simulink model "progetto3Tenzo"  (Simulink 7.9)
settings: Solver=ode23s  StartTime=0.0  StopTime=100  RelTol=1e-3
values from neighbouring files (symbols this model uses):
  AMI = AK1    [AstaTenzo.m]    (also in BoundTenzo.m)
  AMin = [ ... (first row only)    [AstaTenzo.m]    (also in BoundTenzo.m; RiduzioneModello1_15.m)
  Aoss = AMin-V*ClocalMin    [AstaTenzo.m]    (also in BoundTenzo.m; RiduzioneModello1_15.m)
  BMI = BK1    [AstaTenzo.m]    (also in BoundTenzo.m)
  Bmod = [M BMin]    [AstaTenzo.m]    (also in BoundTenzo.m)
  Boss = [BMin-V*D V M-V*N]    [AstaTenzo.m]    (also in BoundTenzo.m; RiduzioneModello1_15.m = [BMin-V*D V])
  ClocalMin = [ ... (first row only)    [AstaTenzo.m]    (also in BoundTenzo.m; RiduzioneModello1_15.m)
  CMI = eye(q*mu)    [AstaTenzo.m]    (also in BoundTenzo.m)
  Coss = eye(n)    [AstaTenzo.m]    (also in BoundTenzo.m; RiduzioneModello1_15.m = eye(size(AMin)))
  DMI = zeros(q*mu,q)    [AstaTenzo.m]    (also in BoundTenzo.m)
  Dmod = [N D]    [AstaTenzo.m]    (also in BoundTenzo.m)
  Doss = zeros(size(Boss))    [AstaTenzo.m]    (also in BoundTenzo.m; RiduzioneModello1_15.m)
  F1 = F(:,size(AMin,1)+1:size(F,2))    [AstaTenzo.m]    (also in BoundTenzo.m)
  F2 = F(:,1:size(AMin,1))    [AstaTenzo.m]    (also in BoundTenzo.m)
  omega = 0.5    [AstaTenzo.m]    (also in BoundTenzo.m = logspace(-2,1,150); LTR_Tenzo.m = logspace(-2,3); Tenzo1_05.m = 4)
libraries: simulink x1
settings Model: Creator=danilo  LastModifiedBy=userk
settings DebuggingCC: FcnCallInpInsideContextMsg=Use local settings
settings GRTTargetCC: CombineOutputUpdateFcns=off  GRTInterface=on

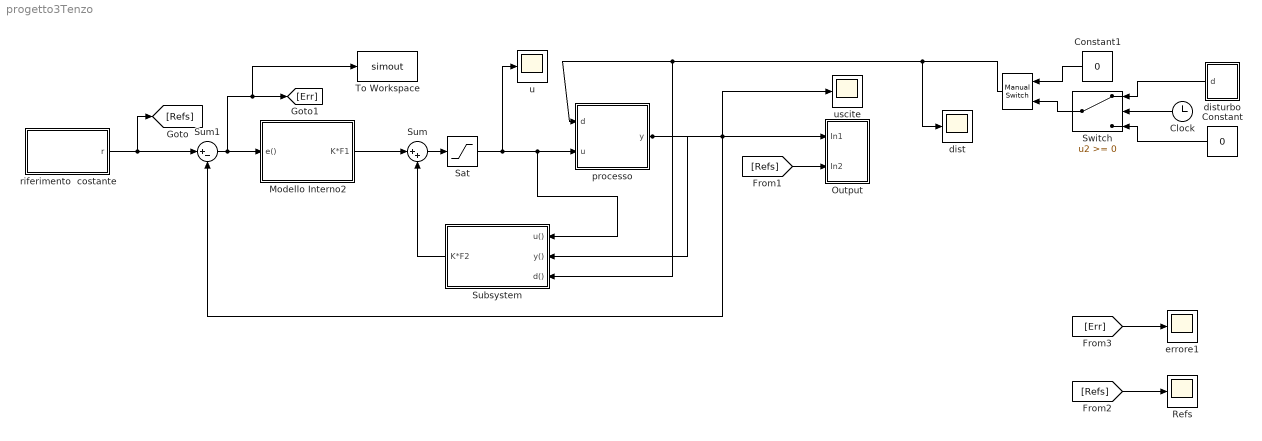
== system progetto3Tenzo ==
  " " : simulink/Signal Routing/Manual Switch  sw=0  action=0  varsize=off
  Clock : Clock
  Constant : Constant  Value=0
  Constant1 : Constant  Value=0
  Modello Interno2 : Subsystem
  Output : Subsystem
  Refs : Scope
  Sat : Saturate  UpperLimit=60  LowerLimit=-60
  Subsystem : Subsystem
  Sum : Sum  Inputs=|++
  Sum1 : Sum  Inputs=|+-
  Switch : Switch
  To Workspace : ToWorkspace  VariableName=simout  SampleTime=-1  SaveFormat=Structure
  dist : Scope
      settings: SaveName=ScopeData5
  disturbo : Subsystem
  errore1 : Scope
      settings: SaveName=ScopeData8
  processo : Subsystem
  riferimento  costante : Subsystem
  u : Scope
      settings: SaveName=ScopeData3
  uscite : Scope
      settings: SaveName=ScopeData2
  wires:
  riferimento  costante/1(r) -> Sum1/1, [Refs]
  processo/1(y) -> Sum1/2, Output/1(In1), uscite/1, Subsystem/2(y())
  Subsystem/1(K*F2) -> Sum/2
  Sum/1 -> Sat/1
  Sum1/1 -> To Workspace/1, [Err], Modello Interno2/1(e())
  [Refs] -> Output/2(In2)
  [Refs] -> Refs/1
  [Err] -> errore1/1
  Clock/1 -> Switch/2
  disturbo/1(d) -> Switch/1
  Constant/1 -> Switch/3
  Sat/1 -> processo/2(u), Subsystem/1(u()), u/1
  Switch/1 -> " "/2
  Constant1/1 -> " "/1
  " "/1 -> dist/1, processo/1(d), Subsystem/3(d())
  Modello Interno2/1(K*F1) -> Sum/1

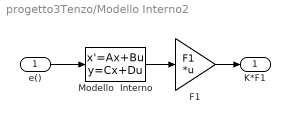
== system progetto3Tenzo/Modello Interno2 ==
  e() : Inport
  F1 : Gain  Gain=F1  Multiplication=Matrix(K*u) (u vector)
  Modello  Interno : StateSpace  A=AMI  B=BMI  C=CMI  D=DMI
  K*F1 : Outport
  wires:
  Modello  Interno/1 -> F1/1
  e()/1 -> Modello  Interno/1
  F1/1 -> K*F1/1

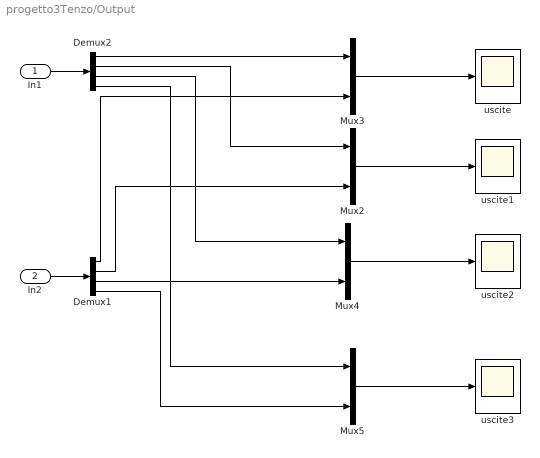
== system progetto3Tenzo/Output ==
  In1 : Inport
  In2 : Inport  Port=2
  Demux1 : Demux
  Demux2 : Demux
  Mux{2..5} (4 alike) : Mux  Inputs=2
  uscite{,1..3} (4 alike) : Scope
      uscite settings: TickLabels=on  YMin=-3.5  YMax=7
      uscite1 settings: TickLabels=on  TimeRange=30  YMin=0.75  YMax=4.25  SaveName=ScopeData4
      uscite2 settings: TickLabels=on  YMin=0.75  YMax=4.25  SaveName=ScopeData6
      uscite3 settings: TickLabels=on  YMin=0.75  YMax=4.25  SaveName=ScopeData7
  wires:
  Demux1/1 -> Mux3/2
  In2/1 -> Demux1/1
  In1/1 -> Demux2/1
  Mux3/1 -> uscite/1
  Demux2/1 -> Mux3/1
  Mux2/1 -> uscite1/1
  Demux2/2 -> Mux2/1
  Mux4/1 -> uscite2/1
  Demux2/3 -> Mux4/1
  Mux5/1 -> uscite3/1
  Demux2/4 -> Mux5/1
  Demux1/2 -> Mux2/2
  Demux1/3 -> Mux4/2
  Demux1/4 -> Mux5/2

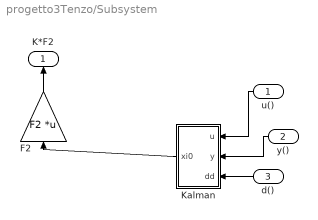
== system progetto3Tenzo/Subsystem ==
  u() : Inport
  y() : Inport  Port=2
  d() : Inport  Port=3
  F2 : Gain  Gain=F2  Multiplication=Matrix(K*u) (u vector)
  Kalman : Subsystem
  K*F2 : Outport
  wires:
  Kalman/1(xi0) -> F2/1
  u()/1 -> Kalman/1(u)
  y()/1 -> Kalman/2(y)
  d()/1 -> Kalman/3(dd)
  F2/1 -> K*F2/1

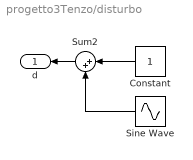
== system progetto3Tenzo/disturbo ==
  Constant : Constant
  Sine Wave : Sin  Amplitude=3  Frequency=omega  SampleTime=0
  Sum2 : Sum  Inputs=|++
  d : Outport
  wires:
  Sine Wave/1 -> Sum2/2
  Constant/1 -> Sum2/1
  Sum2/1 -> d/1

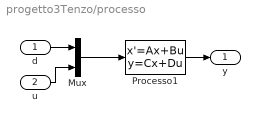
== system progetto3Tenzo/processo ==
  d : Inport
  u : Inport  Port=2
  Mux : Mux  Inputs=[1 4]
  Processo1 : StateSpace  A=AMin  B=Bmod  C=ClocalMin  D=Dmod
  y : Outport
  wires:
  Mux/1 -> Processo1/1
  d/1 -> Mux/1
  Processo1/1 -> y/1
  u/1 -> Mux/2

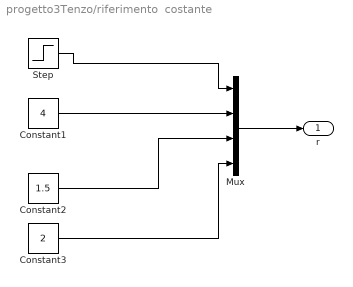
== system progetto3Tenzo/riferimento  costante ==
  Constant1 : Constant  Value=4
  Constant2 : Constant  Value=1.5
  Constant3 : Constant  Value=2
  Mux : Mux  Inputs=[1 1 1 1]
  Step : Step  Time=3  After=2.5  SampleTime=0
  r : Outport
  wires:
  Mux/1 -> r/1
  Step/1 -> Mux/1
  Constant1/1 -> Mux/2
  Constant2/1 -> Mux/3
  Constant3/1 -> Mux/4

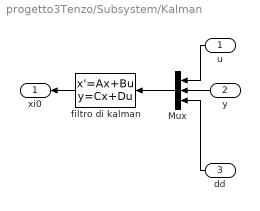
== system progetto3Tenzo/Subsystem/Kalman ==
  u : Inport
  y : Inport  Port=2
  dd : Inport  Port=3
  Mux : Mux  Inputs=[4 4 1]
  filtro di kalman : StateSpace  A=Aoss  B=Boss  C=Coss  D=Doss
  xi0 : Outport
  wires:
  Mux/1 -> filtro di kalman/1
  u/1 -> Mux/1
  filtro di kalman/1 -> xi0/1
  y/1 -> Mux/2
  dd/1 -> Mux/3
